simulink model "OIRT"  (Simulink 8.5)
settings: Solver=ode3  SolverMode=SingleTasking  StartTime=0.0  StopTime=1.0  FixedStep=2e-5  RelTol=1e-4  AbsTol=1e-6
undefined symbols (not defined in the file or in its folder): DAB, den, elements, num
libraries: powerlib x191, powerlib_extras x6
(part 3 of 9)

== system OIRT/Off-Line Analysis/Line 3/Fault ==
  faultA : Inport
  faultB : Inport  Port=2
  faultC : Inport  Port=3
  faultG : Inport  Port=4
  Tfault : Inport  Port=5
  &{,1..3} (4 alike) : Logic
  BreakerA : powerlib/Elements/Breaker  InitialState=0  SwitchingTimes="[ 1/60  5/60 ]"  External=on  BreakerResistance=0.01  SnubberResistance=1e6  SnubberCapacitance=inf  Measurements=None  MoreParameters=off  NoBreakLoop=off
  BreakerB : powerlib/Elements/Breaker  InitialState=0  SwitchingTimes="[ 1/60  5/60 ]"  External=on  BreakerResistance=0.01  SnubberResistance=1e6  SnubberCapacitance=inf  Measurements=None  MoreParameters=off  NoBreakLoop=off
  BreakerC : powerlib/Elements/Breaker  InitialState=0  SwitchingTimes="[ 1/60  5/60 ]"  External=on  BreakerResistance=0.01  SnubberResistance=1e6  SnubberCapacitance=inf  Measurements=None  MoreParameters=off  NoBreakLoop=off
  BreakerN : powerlib/Elements/Breaker  InitialState=0  SwitchingTimes="[ 1/60  5/60 ]"  External=on  BreakerResistance=0.01  SnubberResistance=1e6  SnubberCapacitance=inf  Measurements=None  MoreParameters=off  NoBreakLoop=off
  Ground : powerlib/Elements/Ground  LConnTagsString=a
  RA : powerlib/Elements/Series RLC Branch  LConnTagsString=__new0  RConnTagsString=__new0  BranchType=R  Resistance=10000  Inductance=1e-3  SetiL0=off  InitialCurrent=0  Capacitance=1e-6  Setx0=off  InitialVoltage=0  Measurements=None
  RB : powerlib/Elements/Series RLC Branch  LConnTagsString=__new0  RConnTagsString=__new0  BranchType=R  Resistance=10000  Inductance=1e-3  SetiL0=off  InitialCurrent=0  Capacitance=1e-6  Setx0=off  InitialVoltage=0  Measurements=None
  RC : powerlib/Elements/Series RLC Branch  LConnTagsString=__new0  RConnTagsString=__new0  BranchType=R  Resistance=10000  Inductance=1e-3  SetiL0=off  InitialCurrent=0  Capacitance=1e-6  Setx0=off  InitialVoltage=0  Measurements=None
  RN : powerlib/Elements/Series RLC Branch  LConnTagsString=__new0  RConnTagsString=__new0  BranchType=R  Resistance=10000  Inductance=1e-3  SetiL0=off  InitialCurrent=0  Capacitance=1e-6  Setx0=off  InitialVoltage=0  Measurements=None
  RfA : powerlib/Elements/Series RLC Branch  LConnTagsString=__new0  RConnTagsString=__new0  BranchType=R  Resistance=faultR  Inductance=1e-3  SetiL0=off  InitialCurrent=0  Capacitance=1e-6  Setx0=off  InitialVoltage=0  Measurements=None
  RfB : powerlib/Elements/Series RLC Branch  LConnTagsString=__new0  RConnTagsString=__new0  BranchType=R  Resistance=faultR  Inductance=1e-3  SetiL0=off  InitialCurrent=0  Capacitance=1e-6  Setx0=off  InitialVoltage=0  Measurements=None
  RfC : powerlib/Elements/Series RLC Branch  LConnTagsString=__new0  RConnTagsString=__new0  BranchType=R  Resistance=faultR  Inductance=1e-3  SetiL0=off  InitialCurrent=0  Capacitance=1e-6  Setx0=off  InitialVoltage=0  Measurements=None
  A : PMIOPort  Tag=PMCPort  Port=1  Side=Left
  B : PMIOPort  Tag=PMCPort  Port=2  Side=Left
  C : PMIOPort  Tag=PMCPort  Port=3  Side=Left
  wires:
  &2/1 -> BreakerC/1
  &1/1 -> BreakerB/1
  &/1 -> BreakerA/1
  &3/1 -> BreakerN/1
  Tfault/1 -> &/2, &1/2, &2/2, &3/2
  faultG/1 -> &3/1
  faultC/1 -> &2/1
  faultB/1 -> &1/1
  faultA/1 -> &/1
  connections:
  RN/RConn1 -- Ground/LConn1 -- BreakerN/RConn1
  RfC/RConn1 -- RfA/RConn1 -- RfB/RConn1 -- RN/LConn1 -- BreakerN/LConn1
  BreakerA/RConn1 -- RfA/LConn1 -- RA/RConn1
  BreakerB/RConn1 -- RfB/LConn1 -- RB/RConn1
  RfC/LConn1 -- RC/RConn1 -- BreakerC/RConn1
  BreakerC/LConn1 -- C/RConn1 -- RC/LConn1
  RA/LConn1 -- BreakerA/LConn1 -- A/RConn1
  BreakerB/LConn1 -- RB/LConn1 -- B/RConn1

== system OIRT/Off-Line Analysis/Line 3/Fault Selector ==
  "  " : Constant  Value=faultType
  "  +" : Logic  Operator=OR  Inputs=7
  " +" : Logic  Operator=OR  Inputs=5
  + : Logic  Operator=OR  Inputs=5
  "+ " : Logic  Operator=OR  Inputs=6
  A-B-C : Fcn  Expr=(u(1)==8)
  A-B-C-G : Fcn  Expr=(u(1)==9)
  A-G : Fcn  Expr=(u(1)==1)
  B-C : Fcn  Expr=(u(1)==4)
  B-C-G : Fcn  Expr=(u(1)==5)
  B-G : Fcn  Expr=(u(1)==2)
  C-A : Fcn  Expr=(u(1)==6)
  C-A-G : Fcn  Expr=(u(1)==7)
  C-G : Fcn  Expr=(u(1)==3)
  faultA : Outport  InitialOutput=0
  faultB : Outport  Port=2  InitialOutput=0
  faultC : Outport  Port=3  InitialOutput=0
  faultG : Outport  Port=4  InitialOutput=0
  wires:
  A-B-C/1 -> +/4, "  +"/6, " +"/4
  A-B-C-G/1 -> +/5, "+ "/6, "  +"/7, " +"/5
  C-A-G/1 -> +/3, "+ "/5, "  +"/5
  C-G/1 -> "+ "/3, "  +"/1
  B-C-G/1 -> " +"/3, "+ "/4, "  +"/3
  B-C/1 -> " +"/2, "  +"/2
  B-G/1 -> "+ "/2, " +"/1
  C-A/1 -> +/2, "  +"/4
  A-G/1 -> +/1, "+ "/1
  "+ "/1 -> faultG/1
  "  +"/1 -> faultC/1
  " +"/1 -> faultB/1
  +/1 -> faultA/1
  "  "/1 -> B-C-G/1, A-B-C-G/1, A-B-C/1, C-A-G/1, C-A/1, B-C/1, B-G/1, A-G/1, C-G/1

== system OIRT/On-Line Analysis/Line 1/Fault ==
  faultA : Inport
  faultB : Inport  Port=2
  faultC : Inport  Port=3
  faultG : Inport  Port=4
  Tfault : Inport  Port=5
  &{,1..3} (4 alike) : Logic
  BreakerA : powerlib/Elements/Breaker  InitialState=0  SwitchingTimes="[ 1/60  5/60 ]"  External=on  BreakerResistance=0.01  SnubberResistance=1e6  SnubberCapacitance=inf  Measurements=None  MoreParameters=off  NoBreakLoop=off
  BreakerB : powerlib/Elements/Breaker  InitialState=0  SwitchingTimes="[ 1/60  5/60 ]"  External=on  BreakerResistance=0.01  SnubberResistance=1e6  SnubberCapacitance=inf  Measurements=None  MoreParameters=off  NoBreakLoop=off
  BreakerC : powerlib/Elements/Breaker  InitialState=0  SwitchingTimes="[ 1/60  5/60 ]"  External=on  BreakerResistance=0.01  SnubberResistance=1e6  SnubberCapacitance=inf  Measurements=None  MoreParameters=off  NoBreakLoop=off
  BreakerN : powerlib/Elements/Breaker  InitialState=0  SwitchingTimes="[ 1/60  5/60 ]"  External=on  BreakerResistance=0.01  SnubberResistance=1e6  SnubberCapacitance=inf  Measurements=None  MoreParameters=off  NoBreakLoop=off
  Ground : powerlib/Elements/Ground  LConnTagsString=a
  RA : powerlib/Elements/Series RLC Branch  LConnTagsString=__new0  RConnTagsString=__new0  BranchType=R  Resistance=10000  Inductance=1e-3  SetiL0=off  InitialCurrent=0  Capacitance=1e-6  Setx0=off  InitialVoltage=0  Measurements=None
  RB : powerlib/Elements/Series RLC Branch  LConnTagsString=__new0  RConnTagsString=__new0  BranchType=R  Resistance=10000  Inductance=1e-3  SetiL0=off  InitialCurrent=0  Capacitance=1e-6  Setx0=off  InitialVoltage=0  Measurements=None
  RC : powerlib/Elements/Series RLC Branch  LConnTagsString=__new0  RConnTagsString=__new0  BranchType=R  Resistance=10000  Inductance=1e-3  SetiL0=off  InitialCurrent=0  Capacitance=1e-6  Setx0=off  InitialVoltage=0  Measurements=None
  RN : powerlib/Elements/Series RLC Branch  LConnTagsString=__new0  RConnTagsString=__new0  BranchType=R  Resistance=10000  Inductance=1e-3  SetiL0=off  InitialCurrent=0  Capacitance=1e-6  Setx0=off  InitialVoltage=0  Measurements=None
  RfA : powerlib/Elements/Series RLC Branch  LConnTagsString=__new0  RConnTagsString=__new0  BranchType=R  Resistance=faultR  Inductance=1e-3  SetiL0=off  InitialCurrent=0  Capacitance=1e-6  Setx0=off  InitialVoltage=0  Measurements=None
  RfB : powerlib/Elements/Series RLC Branch  LConnTagsString=__new0  RConnTagsString=__new0  BranchType=R  Resistance=faultR  Inductance=1e-3  SetiL0=off  InitialCurrent=0  Capacitance=1e-6  Setx0=off  InitialVoltage=0  Measurements=None
  RfC : powerlib/Elements/Series RLC Branch  LConnTagsString=__new0  RConnTagsString=__new0  BranchType=R  Resistance=faultR  Inductance=1e-3  SetiL0=off  InitialCurrent=0  Capacitance=1e-6  Setx0=off  InitialVoltage=0  Measurements=None
  A : PMIOPort  Tag=PMCPort  Port=1  Side=Left
  B : PMIOPort  Tag=PMCPort  Port=2  Side=Left
  C : PMIOPort  Tag=PMCPort  Port=3  Side=Left
  wires:
  faultA/1 -> &/1
  faultB/1 -> &1/1
  faultC/1 -> &2/1
  faultG/1 -> &3/1
  Tfault/1 -> &3/2, &2/2, &1/2, &/2
  &3/1 -> BreakerN/1
  &/1 -> BreakerA/1
  &1/1 -> BreakerB/1
  &2/1 -> BreakerC/1
  connections:
  B/RConn1 -- RB/LConn1 -- BreakerB/LConn1
  A/RConn1 -- BreakerA/LConn1 -- RA/LConn1
  RC/LConn1 -- C/RConn1 -- BreakerC/LConn1
  BreakerC/RConn1 -- RC/RConn1 -- RfC/LConn1
  RB/RConn1 -- RfB/LConn1 -- BreakerB/RConn1
  RA/RConn1 -- RfA/LConn1 -- BreakerA/RConn1
  BreakerN/LConn1 -- RN/LConn1 -- RfB/RConn1 -- RfA/RConn1 -- RfC/RConn1
  BreakerN/RConn1 -- Ground/LConn1 -- RN/RConn1

== system OIRT/On-Line Analysis/Line 1/Fault Selector ==
  "  " : Constant  Value=faultType
  "  +" : Logic  Operator=OR  Inputs=7
  " +" : Logic  Operator=OR  Inputs=5
  + : Logic  Operator=OR  Inputs=5
  "+ " : Logic  Operator=OR  Inputs=6
  A-B-C : Fcn  Expr=(u(1)==8)
  A-B-C-G : Fcn  Expr=(u(1)==9)
  A-G : Fcn  Expr=(u(1)==1)
  B-C : Fcn  Expr=(u(1)==4)
  B-C-G : Fcn  Expr=(u(1)==5)
  B-G : Fcn  Expr=(u(1)==2)
  C-A : Fcn  Expr=(u(1)==6)
  C-A-G : Fcn  Expr=(u(1)==7)
  C-G : Fcn  Expr=(u(1)==3)
  faultA : Outport  InitialOutput=0
  faultB : Outport  Port=2  InitialOutput=0
  faultC : Outport  Port=3  InitialOutput=0
  faultG : Outport  Port=4  InitialOutput=0
  wires:
  "  "/1 -> C-G/1, A-G/1, B-G/1, B-C/1, C-A/1, C-A-G/1, A-B-C/1, A-B-C-G/1, B-C-G/1
  +/1 -> faultA/1
  " +"/1 -> faultB/1
  "  +"/1 -> faultC/1
  "+ "/1 -> faultG/1
  A-G/1 -> "+ "/1, +/1
  C-A/1 -> "  +"/4, +/2
  B-G/1 -> " +"/1, "+ "/2
  B-C/1 -> "  +"/2, " +"/2
  B-C-G/1 -> "  +"/3, "+ "/4, " +"/3
  C-G/1 -> "  +"/1, "+ "/3
  C-A-G/1 -> "  +"/5, "+ "/5, +/3
  A-B-C-G/1 -> " +"/5, "  +"/7, "+ "/6, +/5
  A-B-C/1 -> " +"/4, "  +"/6, +/4

== system OIRT/On-Line Analysis/Line 2/Fault ==
  faultA : Inport
  faultB : Inport  Port=2
  faultC : Inport  Port=3
  faultG : Inport  Port=4
  Tfault : Inport  Port=5
  &{,1..3} (4 alike) : Logic
  BreakerA : powerlib/Elements/Breaker  InitialState=0  SwitchingTimes="[ 1/60  5/60 ]"  External=on  BreakerResistance=0.01  SnubberResistance=1e6  SnubberCapacitance=inf  Measurements=None  MoreParameters=off  NoBreakLoop=off
  BreakerB : powerlib/Elements/Breaker  InitialState=0  SwitchingTimes="[ 1/60  5/60 ]"  External=on  BreakerResistance=0.01  SnubberResistance=1e6  SnubberCapacitance=inf  Measurements=None  MoreParameters=off  NoBreakLoop=off
  BreakerC : powerlib/Elements/Breaker  InitialState=0  SwitchingTimes="[ 1/60  5/60 ]"  External=on  BreakerResistance=0.01  SnubberResistance=1e6  SnubberCapacitance=inf  Measurements=None  MoreParameters=off  NoBreakLoop=off
  BreakerN : powerlib/Elements/Breaker  InitialState=0  SwitchingTimes="[ 1/60  5/60 ]"  External=on  BreakerResistance=0.01  SnubberResistance=1e6  SnubberCapacitance=inf  Measurements=None  MoreParameters=off  NoBreakLoop=off
  Ground : powerlib/Elements/Ground  LConnTagsString=a
  RA : powerlib/Elements/Series RLC Branch  LConnTagsString=__new0  RConnTagsString=__new0  BranchType=R  Resistance=10000  Inductance=1e-3  SetiL0=off  InitialCurrent=0  Capacitance=1e-6  Setx0=off  InitialVoltage=0  Measurements=None
  RB : powerlib/Elements/Series RLC Branch  LConnTagsString=__new0  RConnTagsString=__new0  BranchType=R  Resistance=10000  Inductance=1e-3  SetiL0=off  InitialCurrent=0  Capacitance=1e-6  Setx0=off  InitialVoltage=0  Measurements=None
  RC : powerlib/Elements/Series RLC Branch  LConnTagsString=__new0  RConnTagsString=__new0  BranchType=R  Resistance=10000  Inductance=1e-3  SetiL0=off  InitialCurrent=0  Capacitance=1e-6  Setx0=off  InitialVoltage=0  Measurements=None
  RN : powerlib/Elements/Series RLC Branch  LConnTagsString=__new0  RConnTagsString=__new0  BranchType=R  Resistance=10000  Inductance=1e-3  SetiL0=off  InitialCurrent=0  Capacitance=1e-6  Setx0=off  InitialVoltage=0  Measurements=None
  RfA : powerlib/Elements/Series RLC Branch  LConnTagsString=__new0  RConnTagsString=__new0  BranchType=R  Resistance=faultR  Inductance=1e-3  SetiL0=off  InitialCurrent=0  Capacitance=1e-6  Setx0=off  InitialVoltage=0  Measurements=None
  RfB : powerlib/Elements/Series RLC Branch  LConnTagsString=__new0  RConnTagsString=__new0  BranchType=R  Resistance=faultR  Inductance=1e-3  SetiL0=off  InitialCurrent=0  Capacitance=1e-6  Setx0=off  InitialVoltage=0  Measurements=None
  RfC : powerlib/Elements/Series RLC Branch  LConnTagsString=__new0  RConnTagsString=__new0  BranchType=R  Resistance=faultR  Inductance=1e-3  SetiL0=off  InitialCurrent=0  Capacitance=1e-6  Setx0=off  InitialVoltage=0  Measurements=None
  A : PMIOPort  Tag=PMCPort  Port=1  Side=Left
  B : PMIOPort  Tag=PMCPort  Port=2  Side=Left
  C : PMIOPort  Tag=PMCPort  Port=3  Side=Left
  wires:
  faultA/1 -> &/1
  faultB/1 -> &1/1
  faultC/1 -> &2/1
  faultG/1 -> &3/1
  Tfault/1 -> &3/2, &2/2, &1/2, &/2
  &3/1 -> BreakerN/1
  &/1 -> BreakerA/1
  &1/1 -> BreakerB/1
  &2/1 -> BreakerC/1
  connections:
  B/RConn1 -- RB/LConn1 -- BreakerB/LConn1
  A/RConn1 -- BreakerA/LConn1 -- RA/LConn1
  RC/LConn1 -- C/RConn1 -- BreakerC/LConn1
  BreakerC/RConn1 -- RC/RConn1 -- RfC/LConn1
  RB/RConn1 -- RfB/LConn1 -- BreakerB/RConn1
  RA/RConn1 -- RfA/LConn1 -- BreakerA/RConn1
  BreakerN/LConn1 -- RN/LConn1 -- RfB/RConn1 -- RfA/RConn1 -- RfC/RConn1
  BreakerN/RConn1 -- Ground/LConn1 -- RN/RConn1

== system OIRT/On-Line Analysis/Line 2/Fault Selector ==
  "  " : Constant  Value=faultType
  "  +" : Logic  Operator=OR  Inputs=7
  " +" : Logic  Operator=OR  Inputs=5
  + : Logic  Operator=OR  Inputs=5
  "+ " : Logic  Operator=OR  Inputs=6
  A-B-C : Fcn  Expr=(u(1)==8)
  A-B-C-G : Fcn  Expr=(u(1)==9)
  A-G : Fcn  Expr=(u(1)==1)
  B-C : Fcn  Expr=(u(1)==4)
  B-C-G : Fcn  Expr=(u(1)==5)
  B-G : Fcn  Expr=(u(1)==2)
  C-A : Fcn  Expr=(u(1)==6)
  C-A-G : Fcn  Expr=(u(1)==7)
  C-G : Fcn  Expr=(u(1)==3)
  faultA : Outport  InitialOutput=0
  faultB : Outport  Port=2  InitialOutput=0
  faultC : Outport  Port=3  InitialOutput=0
  faultG : Outport  Port=4  InitialOutput=0
  wires:
  "  "/1 -> C-G/1, A-G/1, B-G/1, B-C/1, C-A/1, C-A-G/1, A-B-C/1, A-B-C-G/1, B-C-G/1
  +/1 -> faultA/1
  " +"/1 -> faultB/1
  "  +"/1 -> faultC/1
  "+ "/1 -> faultG/1
  A-G/1 -> "+ "/1, +/1
  C-A/1 -> "  +"/4, +/2
  B-G/1 -> " +"/1, "+ "/2
  B-C/1 -> "  +"/2, " +"/2
  B-C-G/1 -> "  +"/3, "+ "/4, " +"/3
  C-G/1 -> "  +"/1, "+ "/3
  C-A-G/1 -> "  +"/5, "+ "/5, +/3
  A-B-C-G/1 -> " +"/5, "  +"/7, "+ "/6, +/5
  A-B-C/1 -> " +"/4, "  +"/6, +/4

== system OIRT/On-Line Analysis/Line 3/Fault ==
  faultA : Inport
  faultB : Inport  Port=2
  faultC : Inport  Port=3
  faultG : Inport  Port=4
  Tfault : Inport  Port=5
  &{,1..3} (4 alike) : Logic
  BreakerA : powerlib/Elements/Breaker  InitialState=0  SwitchingTimes="[ 1/60  5/60 ]"  External=on  BreakerResistance=0.01  SnubberResistance=1e6  SnubberCapacitance=inf  Measurements=None  MoreParameters=off  NoBreakLoop=off
  BreakerB : powerlib/Elements/Breaker  InitialState=0  SwitchingTimes="[ 1/60  5/60 ]"  External=on  BreakerResistance=0.01  SnubberResistance=1e6  SnubberCapacitance=inf  Measurements=None  MoreParameters=off  NoBreakLoop=off
  BreakerC : powerlib/Elements/Breaker  InitialState=0  SwitchingTimes="[ 1/60  5/60 ]"  External=on  BreakerResistance=0.01  SnubberResistance=1e6  SnubberCapacitance=inf  Measurements=None  MoreParameters=off  NoBreakLoop=off
  BreakerN : powerlib/Elements/Breaker  InitialState=0  SwitchingTimes="[ 1/60  5/60 ]"  External=on  BreakerResistance=0.01  SnubberResistance=1e6  SnubberCapacitance=inf  Measurements=None  MoreParameters=off  NoBreakLoop=off
  Ground : powerlib/Elements/Ground  LConnTagsString=a
  RA : powerlib/Elements/Series RLC Branch  LConnTagsString=__new0  RConnTagsString=__new0  BranchType=R  Resistance=10000  Inductance=1e-3  SetiL0=off  InitialCurrent=0  Capacitance=1e-6  Setx0=off  InitialVoltage=0  Measurements=None
  RB : powerlib/Elements/Series RLC Branch  LConnTagsString=__new0  RConnTagsString=__new0  BranchType=R  Resistance=10000  Inductance=1e-3  SetiL0=off  InitialCurrent=0  Capacitance=1e-6  Setx0=off  InitialVoltage=0  Measurements=None
  RC : powerlib/Elements/Series RLC Branch  LConnTagsString=__new0  RConnTagsString=__new0  BranchType=R  Resistance=10000  Inductance=1e-3  SetiL0=off  InitialCurrent=0  Capacitance=1e-6  Setx0=off  InitialVoltage=0  Measurements=None
  RN : powerlib/Elements/Series RLC Branch  LConnTagsString=__new0  RConnTagsString=__new0  BranchType=R  Resistance=10000  Inductance=1e-3  SetiL0=off  InitialCurrent=0  Capacitance=1e-6  Setx0=off  InitialVoltage=0  Measurements=None
  RfA : powerlib/Elements/Series RLC Branch  LConnTagsString=__new0  RConnTagsString=__new0  BranchType=R  Resistance=faultR  Inductance=1e-3  SetiL0=off  InitialCurrent=0  Capacitance=1e-6  Setx0=off  InitialVoltage=0  Measurements=None
  RfB : powerlib/Elements/Series RLC Branch  LConnTagsString=__new0  RConnTagsString=__new0  BranchType=R  Resistance=faultR  Inductance=1e-3  SetiL0=off  InitialCurrent=0  Capacitance=1e-6  Setx0=off  InitialVoltage=0  Measurements=None
  RfC : powerlib/Elements/Series RLC Branch  LConnTagsString=__new0  RConnTagsString=__new0  BranchType=R  Resistance=faultR  Inductance=1e-3  SetiL0=off  InitialCurrent=0  Capacitance=1e-6  Setx0=off  InitialVoltage=0  Measurements=None
  A : PMIOPort  Tag=PMCPort  Port=1  Side=Left
  B : PMIOPort  Tag=PMCPort  Port=2  Side=Left
  C : PMIOPort  Tag=PMCPort  Port=3  Side=Left
  wires:
  &2/1 -> BreakerC/1
  &1/1 -> BreakerB/1
  &/1 -> BreakerA/1
  &3/1 -> BreakerN/1
  Tfault/1 -> &/2, &1/2, &2/2, &3/2
  faultG/1 -> &3/1
  faultC/1 -> &2/1
  faultB/1 -> &1/1
  faultA/1 -> &/1
  connections:
  RN/RConn1 -- Ground/LConn1 -- BreakerN/RConn1
  RfC/RConn1 -- RfA/RConn1 -- RfB/RConn1 -- RN/LConn1 -- BreakerN/LConn1
  BreakerA/RConn1 -- RfA/LConn1 -- RA/RConn1
  BreakerB/RConn1 -- RfB/LConn1 -- RB/RConn1
  RfC/LConn1 -- RC/RConn1 -- BreakerC/RConn1
  BreakerC/LConn1 -- C/RConn1 -- RC/LConn1
  RA/LConn1 -- BreakerA/LConn1 -- A/RConn1
  BreakerB/LConn1 -- RB/LConn1 -- B/RConn1

== system OIRT/On-Line Analysis/Line 3/Fault Selector ==
  "  " : Constant  Value=faultType
  "  +" : Logic  Operator=OR  Inputs=7
  " +" : Logic  Operator=OR  Inputs=5
  + : Logic  Operator=OR  Inputs=5
  "+ " : Logic  Operator=OR  Inputs=6
  A-B-C : Fcn  Expr=(u(1)==8)
  A-B-C-G : Fcn  Expr=(u(1)==9)
  A-G : Fcn  Expr=(u(1)==1)
  B-C : Fcn  Expr=(u(1)==4)
  B-C-G : Fcn  Expr=(u(1)==5)
  B-G : Fcn  Expr=(u(1)==2)
  C-A : Fcn  Expr=(u(1)==6)
  C-A-G : Fcn  Expr=(u(1)==7)
  C-G : Fcn  Expr=(u(1)==3)
  faultA : Outport  InitialOutput=0
  faultB : Outport  Port=2  InitialOutput=0
  faultC : Outport  Port=3  InitialOutput=0
  faultG : Outport  Port=4  InitialOutput=0
  wires:
  A-B-C/1 -> +/4, "  +"/6, " +"/4
  A-B-C-G/1 -> +/5, "+ "/6, "  +"/7, " +"/5
  C-A-G/1 -> +/3, "+ "/5, "  +"/5
  C-G/1 -> "+ "/3, "  +"/1
  B-C-G/1 -> " +"/3, "+ "/4, "  +"/3
  B-C/1 -> " +"/2, "  +"/2
  B-G/1 -> "+ "/2, " +"/1
  C-A/1 -> +/2, "  +"/4
  A-G/1 -> +/1, "+ "/1
  "+ "/1 -> faultG/1
  "  +"/1 -> faultC/1
  " +"/1 -> faultB/1
  +/1 -> faultA/1
  "  "/1 -> B-C-G/1, A-B-C-G/1, A-B-C/1, C-A-G/1, C-A/1, B-C/1, B-G/1, A-G/1, C-G/1

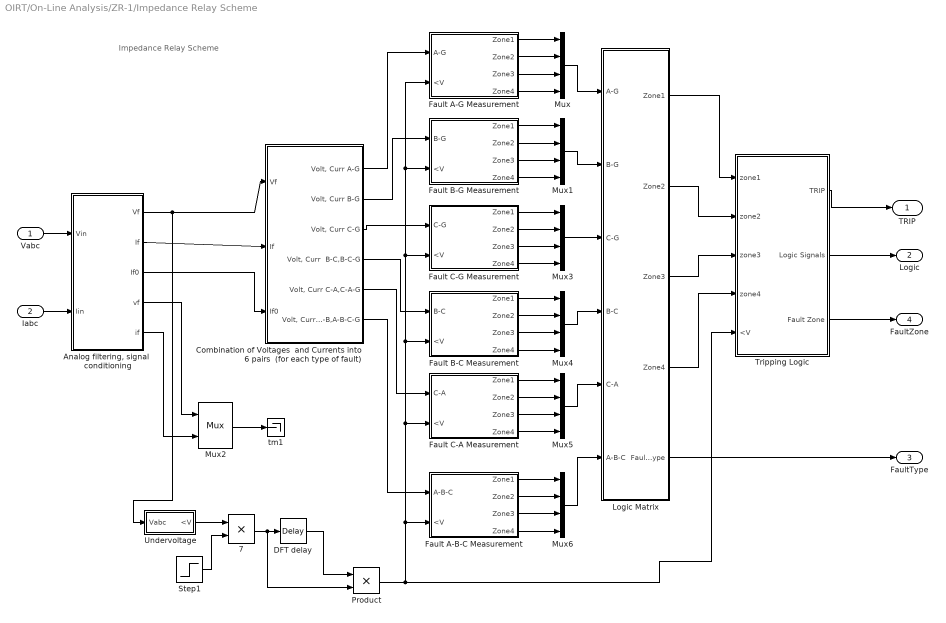
== system OIRT/On-Line Analysis/ZR-1/Impedance Relay Scheme ==
  note: Impedance Relay Scheme
  Vabc : Inport
  Iabc : Inport  Port=2
  " 7" : Product  RndMeth=Zero
  "Analog filtering, signal  conditioning" : Subsystem
  Combination of Voltages  and Currents into 6 pairs  (for each type of fault) : Subsystem
  DFT delay : TransportDelay  DelayTime=0.017  BufferSize=30720
  Fault A-B-C Measurement : Subsystem
  Fault A-G Measurement : Subsystem
  Fault B-C Measurement : Subsystem
  Fault B-G Measurement : Subsystem
  Fault C-A Measurement : Subsystem
  Fault C-G Measurement : Subsystem
  Logic Matrix : Subsystem
  Mux{,1,3..6} (6 alike) : Mux
  Mux2 : Mux  Inputs=2
  Product : Product  RndMeth=Zero
  Step1 : Step  Time=0.017  SampleTime=0
  Tripping Logic : Subsystem
  Undervoltage : Subsystem
  tm1 : Terminator
  "TRIP " : Outport  InitialOutput=0
  Logic : Outport  Port=2  InitialOutput=0
  FaultType : Outport  Port=3  InitialOutput=0
  FaultZone : Outport  Port=4  InitialOutput=0
  wires:
  Mux2/1 -> tm1/1
  Tripping Logic/3(Fault Zone) -> FaultZone/1
  Product/1 -> Tripping Logic/5(<V), Fault A-B-C Measurement/2(<V), Fault C-A Measurement/2(<V), Fault B-C Measurement/2(<V), Fault C-G Measurement/2(<V), Fault B-G Measurement/2(<V), Fault A-G Measurement/2(<V)
  Logic Matrix/5(Fault Type) -> FaultType/1
  Tripping Logic/2(Logic Signals) -> Logic/1
  Tripping Logic/1(TRIP) -> "TRIP "/1
  Logic Matrix/4(" Zone4") -> Tripping Logic/4(zone4)
  Logic Matrix/3(" Zone3") -> Tripping Logic/3(zone3)
  Logic Matrix/2(" Zone2") -> Tripping Logic/2(zone2)
  Logic Matrix/1(" Zone1") -> Tripping Logic/1(zone1)
  Mux6/1 -> Logic Matrix/6(A-B-C)
  Mux5/1 -> Logic Matrix/5(C-A)
  Mux4/1 -> Logic Matrix/4(B-C)
  Mux3/1 -> Logic Matrix/3(C-G)
  Mux1/1 -> Logic Matrix/2(B-G)
  Mux/1 -> Logic Matrix/1(A-G)
  Fault A-B-C Measurement/4(Zone4) -> Mux6/4
  Fault A-B-C Measurement/3(Zone3) -> Mux6/3
  Fault A-B-C Measurement/2(Zone2) -> Mux6/2
  Fault A-B-C Measurement/1(Zone1) -> Mux6/1
  Fault C-A Measurement/4(Zone4) -> Mux5/4
  Fault C-A Measurement/3(Zone3) -> Mux5/3
  Fault C-A Measurement/2(Zone2) -> Mux5/2
  Fault C-A Measurement/1(Zone1) -> Mux5/1
  Fault B-C Measurement/4(Zone4) -> Mux4/4
  Fault B-C Measurement/3(Zone3) -> Mux4/3
  Fault B-C Measurement/2(Zone2) -> Mux4/2
  Fault B-C Measurement/1(Zone1) -> Mux4/1
  Fault C-G Measurement/4(Zone4) -> Mux3/4
  Fault C-G Measurement/3(Zone3) -> Mux3/3
  Fault C-G Measurement/2(Zone2) -> Mux3/2
  Fault C-G Measurement/1(Zone1) -> Mux3/1
  Fault B-G Measurement/4(Zone4) -> Mux1/4
  Fault B-G Measurement/3(Zone3) -> Mux1/3
  Fault B-G Measurement/2(Zone2) -> Mux1/2
  Fault B-G Measurement/1(Zone1) -> Mux1/1
  Fault A-G Measurement/4(Zone4) -> Mux/4
  Fault A-G Measurement/3(Zone3) -> Mux/3
  Fault A-G Measurement/2(Zone2) -> Mux/2
  Fault A-G Measurement/1(Zone1) -> Mux/1
  DFT delay/1 -> Product/1
  Combination of Voltages  and Currents into 6 pairs  (for each type of fault)/6("Volt, Curr A-B,A-B-C-G") -> Fault A-B-C Measurement/1(A-B-C)
  Combination of Voltages  and Currents into 6 pairs  (for each type of fault)/5("Volt, Curr C-A,C-A-G") -> Fault C-A Measurement/1(C-A)
  Combination of Voltages  and Currents into 6 pairs  (for each type of fault)/4("Volt, Curr  B-C,B-C-G") -> Fault B-C Measurement/1(B-C)
  Combination of Voltages  and Currents into 6 pairs  (for each type of fault)/3("Volt, Curr C-G") -> Fault C-G Measurement/1(C-G)
  Combination of Voltages  and Currents into 6 pairs  (for each type of fault)/2("Volt, Curr B-G") -> Fault B-G Measurement/1(B-G)
  "Analog filtering, signal  conditioning"/3(If0) -> Combination of Voltages  and Currents into 6 pairs  (for each type of fault)/3(If0)
  "Analog filtering, signal  conditioning"/2(If) -> Combination of Voltages  and Currents into 6 pairs  (for each type of fault)/2(If)
  "Analog filtering, signal  conditioning"/5(if) -> Mux2/2
  "Analog filtering, signal  conditioning"/4(vf) -> Mux2/1
  "Analog filtering, signal  conditioning"/1(Vf) -> Undervoltage/1("Vabc  "), Combination of Voltages  and Currents into 6 pairs  (for each type of fault)/1(Vf)
  " 7"/1 -> Product/2, DFT delay/1
  Step1/1 -> " 7"/2
  Undervoltage/1(<V) -> " 7"/1
  Combination of Voltages  and Currents into 6 pairs  (for each type of fault)/1("Volt, Curr A-G") -> Fault A-G Measurement/1(A-G)
  Iabc/1 -> "Analog filtering, signal  conditioning"/2(Iin)
  Vabc/1 -> "Analog filtering, signal  conditioning"/1(Vin)

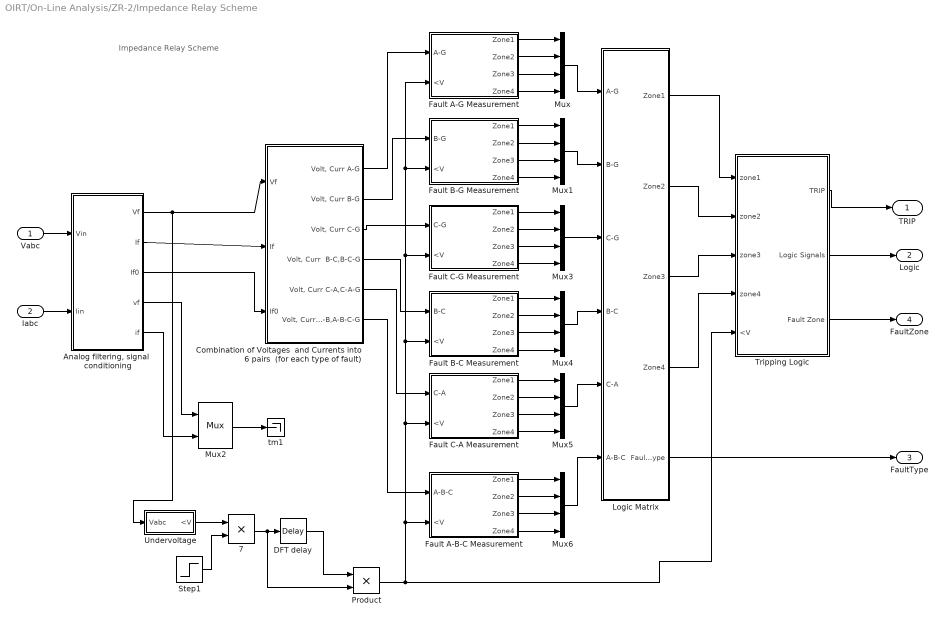
== system OIRT/On-Line Analysis/ZR-2/Impedance Relay Scheme ==
  note: Impedance Relay Scheme
  Vabc : Inport
  Iabc : Inport  Port=2
  " 7" : Product  RndMeth=Zero
  "Analog filtering, signal  conditioning" : Subsystem
  Combination of Voltages  and Currents into 6 pairs  (for each type of fault) : Subsystem
  DFT delay : TransportDelay  DelayTime=0.017  BufferSize=30720
  Fault A-B-C Measurement : Subsystem
  Fault A-G Measurement : Subsystem
  Fault B-C Measurement : Subsystem
  Fault B-G Measurement : Subsystem
  Fault C-A Measurement : Subsystem
  Fault C-G Measurement : Subsystem
  Logic Matrix : Subsystem
  Mux{,1,3..6} (6 alike) : Mux
  Mux2 : Mux  Inputs=2
  Product : Product  RndMeth=Zero
  Step1 : Step  Time=0.017  SampleTime=0
  Tripping Logic : Subsystem
  Undervoltage : Subsystem
  tm1 : Terminator
  "TRIP " : Outport  InitialOutput=0
  Logic : Outport  Port=2  InitialOutput=0
  FaultType : Outport  Port=3  InitialOutput=0
  FaultZone : Outport  Port=4  InitialOutput=0
  wires:
  Mux2/1 -> tm1/1
  Tripping Logic/3(Fault Zone) -> FaultZone/1
  Product/1 -> Tripping Logic/5(<V), Fault A-B-C Measurement/2(<V), Fault C-A Measurement/2(<V), Fault B-C Measurement/2(<V), Fault C-G Measurement/2(<V), Fault B-G Measurement/2(<V), Fault A-G Measurement/2(<V)
  Logic Matrix/5(Fault Type) -> FaultType/1
  Tripping Logic/2(Logic Signals) -> Logic/1
  Tripping Logic/1(TRIP) -> "TRIP "/1
  Logic Matrix/4(" Zone4") -> Tripping Logic/4(zone4)
  Logic Matrix/3(" Zone3") -> Tripping Logic/3(zone3)
  Logic Matrix/2(" Zone2") -> Tripping Logic/2(zone2)
  Logic Matrix/1(" Zone1") -> Tripping Logic/1(zone1)
  Mux6/1 -> Logic Matrix/6(A-B-C)
  Mux5/1 -> Logic Matrix/5(C-A)
  Mux4/1 -> Logic Matrix/4(B-C)
  Mux3/1 -> Logic Matrix/3(C-G)
  Mux1/1 -> Logic Matrix/2(B-G)
  Mux/1 -> Logic Matrix/1(A-G)
  Fault A-B-C Measurement/4(Zone4) -> Mux6/4
  Fault A-B-C Measurement/3(Zone3) -> Mux6/3
  Fault A-B-C Measurement/2(Zone2) -> Mux6/2
  Fault A-B-C Measurement/1(Zone1) -> Mux6/1
  Fault C-A Measurement/4(Zone4) -> Mux5/4
  Fault C-A Measurement/3(Zone3) -> Mux5/3
  Fault C-A Measurement/2(Zone2) -> Mux5/2
  Fault C-A Measurement/1(Zone1) -> Mux5/1
  Fault B-C Measurement/4(Zone4) -> Mux4/4
  Fault B-C Measurement/3(Zone3) -> Mux4/3
  Fault B-C Measurement/2(Zone2) -> Mux4/2
  Fault B-C Measurement/1(Zone1) -> Mux4/1
  Fault C-G Measurement/4(Zone4) -> Mux3/4
  Fault C-G Measurement/3(Zone3) -> Mux3/3
  Fault C-G Measurement/2(Zone2) -> Mux3/2
  Fault C-G Measurement/1(Zone1) -> Mux3/1
  Fault B-G Measurement/4(Zone4) -> Mux1/4
  Fault B-G Measurement/3(Zone3) -> Mux1/3
  Fault B-G Measurement/2(Zone2) -> Mux1/2
  Fault B-G Measurement/1(Zone1) -> Mux1/1
  Fault A-G Measurement/4(Zone4) -> Mux/4
  Fault A-G Measurement/3(Zone3) -> Mux/3
  Fault A-G Measurement/2(Zone2) -> Mux/2
  Fault A-G Measurement/1(Zone1) -> Mux/1
  DFT delay/1 -> Product/1
  Combination of Voltages  and Currents into 6 pairs  (for each type of fault)/6("Volt, Curr A-B,A-B-C-G") -> Fault A-B-C Measurement/1(A-B-C)
  Combination of Voltages  and Currents into 6 pairs  (for each type of fault)/5("Volt, Curr C-A,C-A-G") -> Fault C-A Measurement/1(C-A)
  Combination of Voltages  and Currents into 6 pairs  (for each type of fault)/4("Volt, Curr  B-C,B-C-G") -> Fault B-C Measurement/1(B-C)
  Combination of Voltages  and Currents into 6 pairs  (for each type of fault)/3("Volt, Curr C-G") -> Fault C-G Measurement/1(C-G)
  Combination of Voltages  and Currents into 6 pairs  (for each type of fault)/2("Volt, Curr B-G") -> Fault B-G Measurement/1(B-G)
  "Analog filtering, signal  conditioning"/3(If0) -> Combination of Voltages  and Currents into 6 pairs  (for each type of fault)/3(If0)
  "Analog filtering, signal  conditioning"/2(If) -> Combination of Voltages  and Currents into 6 pairs  (for each type of fault)/2(If)
  "Analog filtering, signal  conditioning"/5(if) -> Mux2/2
  "Analog filtering, signal  conditioning"/4(vf) -> Mux2/1
  "Analog filtering, signal  conditioning"/1(Vf) -> Undervoltage/1("Vabc  "), Combination of Voltages  and Currents into 6 pairs  (for each type of fault)/1(Vf)
  " 7"/1 -> Product/2, DFT delay/1
  Step1/1 -> " 7"/2
  Undervoltage/1(<V) -> " 7"/1
  Combination of Voltages  and Currents into 6 pairs  (for each type of fault)/1("Volt, Curr A-G") -> Fault A-G Measurement/1(A-G)
  Iabc/1 -> "Analog filtering, signal  conditioning"/2(Iin)
  Vabc/1 -> "Analog filtering, signal  conditioning"/1(Vin)

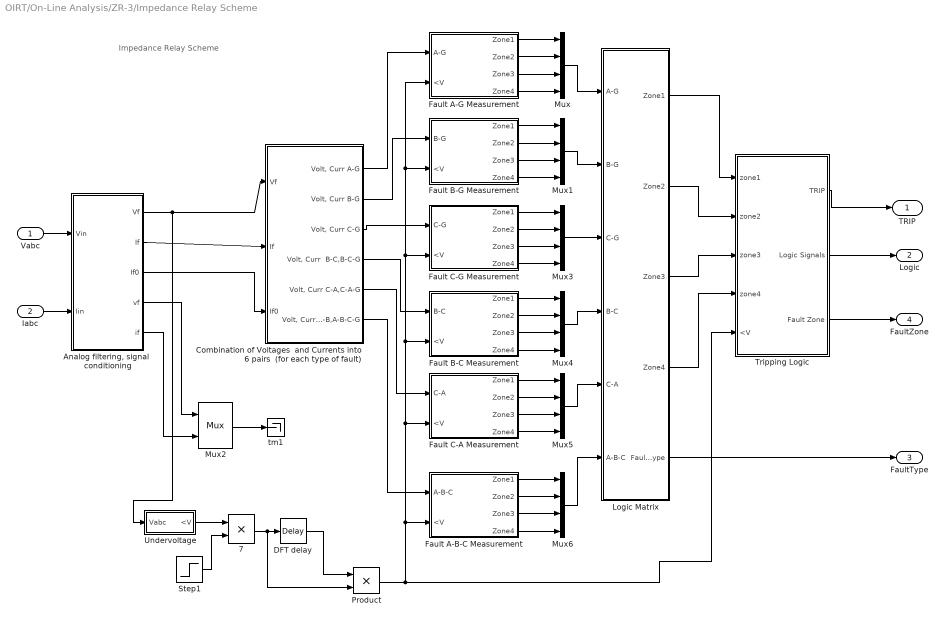
== system OIRT/On-Line Analysis/ZR-3/Impedance Relay Scheme ==
  note: Impedance Relay Scheme
  Vabc : Inport
  Iabc : Inport  Port=2
  " 7" : Product  RndMeth=Zero
  "Analog filtering, signal  conditioning" : Subsystem
  Combination of Voltages  and Currents into 6 pairs  (for each type of fault) : Subsystem
  DFT delay : TransportDelay  DelayTime=0.017  BufferSize=30720
  Fault A-B-C Measurement : Subsystem
  Fault A-G Measurement : Subsystem
  Fault B-C Measurement : Subsystem
  Fault B-G Measurement : Subsystem
  Fault C-A Measurement : Subsystem
  Fault C-G Measurement : Subsystem
  Logic Matrix : Subsystem
  Mux{,1,3..6} (6 alike) : Mux
  Mux2 : Mux  Inputs=2
  Product : Product  RndMeth=Zero
  Step1 : Step  Time=0.017  SampleTime=0
  Tripping Logic : Subsystem
  Undervoltage : Subsystem
  tm1 : Terminator
  "TRIP " : Outport  InitialOutput=0
  Logic : Outport  Port=2  InitialOutput=0
  FaultType : Outport  Port=3  InitialOutput=0
  FaultZone : Outport  Port=4  InitialOutput=0
  wires:
  Vabc/1 -> "Analog filtering, signal  conditioning"/1(Vin)
  Iabc/1 -> "Analog filtering, signal  conditioning"/2(Iin)
  Combination of Voltages  and Currents into 6 pairs  (for each type of fault)/1("Volt, Curr A-G") -> Fault A-G Measurement/1(A-G)
  Undervoltage/1(<V) -> " 7"/1
  Step1/1 -> " 7"/2
  " 7"/1 -> DFT delay/1, Product/2
  "Analog filtering, signal  conditioning"/1(Vf) -> Combination of Voltages  and Currents into 6 pairs  (for each type of fault)/1(Vf), Undervoltage/1("Vabc  ")
  "Analog filtering, signal  conditioning"/4(vf) -> Mux2/1
  "Analog filtering, signal  conditioning"/5(if) -> Mux2/2
  "Analog filtering, signal  conditioning"/2(If) -> Combination of Voltages  and Currents into 6 pairs  (for each type of fault)/2(If)
  "Analog filtering, signal  conditioning"/3(If0) -> Combination of Voltages  and Currents into 6 pairs  (for each type of fault)/3(If0)
  Combination of Voltages  and Currents into 6 pairs  (for each type of fault)/2("Volt, Curr B-G") -> Fault B-G Measurement/1(B-G)
  Combination of Voltages  and Currents into 6 pairs  (for each type of fault)/3("Volt, Curr C-G") -> Fault C-G Measurement/1(C-G)
  Combination of Voltages  and Currents into 6 pairs  (for each type of fault)/4("Volt, Curr  B-C,B-C-G") -> Fault B-C Measurement/1(B-C)
  Combination of Voltages  and Currents into 6 pairs  (for each type of fault)/5("Volt, Curr C-A,C-A-G") -> Fault C-A Measurement/1(C-A)
  Combination of Voltages  and Currents into 6 pairs  (for each type of fault)/6("Volt, Curr A-B,A-B-C-G") -> Fault A-B-C Measurement/1(A-B-C)
  DFT delay/1 -> Product/1
  Fault A-G Measurement/1(Zone1) -> Mux/1
  Fault A-G Measurement/2(Zone2) -> Mux/2
  Fault A-G Measurement/3(Zone3) -> Mux/3
  Fault A-G Measurement/4(Zone4) -> Mux/4
  Fault B-G Measurement/1(Zone1) -> Mux1/1
  Fault B-G Measurement/2(Zone2) -> Mux1/2
  Fault B-G Measurement/3(Zone3) -> Mux1/3
  Fault B-G Measurement/4(Zone4) -> Mux1/4
  Fault C-G Measurement/1(Zone1) -> Mux3/1
  Fault C-G Measurement/2(Zone2) -> Mux3/2
  Fault C-G Measurement/3(Zone3) -> Mux3/3
  Fault C-G Measurement/4(Zone4) -> Mux3/4
  Fault B-C Measurement/1(Zone1) -> Mux4/1
  Fault B-C Measurement/2(Zone2) -> Mux4/2
  Fault B-C Measurement/3(Zone3) -> Mux4/3
  Fault B-C Measurement/4(Zone4) -> Mux4/4
  Fault C-A Measurement/1(Zone1) -> Mux5/1
  Fault C-A Measurement/2(Zone2) -> Mux5/2
  Fault C-A Measurement/3(Zone3) -> Mux5/3
  Fault C-A Measurement/4(Zone4) -> Mux5/4
  Fault A-B-C Measurement/1(Zone1) -> Mux6/1
  Fault A-B-C Measurement/2(Zone2) -> Mux6/2
  Fault A-B-C Measurement/3(Zone3) -> Mux6/3
  Fault A-B-C Measurement/4(Zone4) -> Mux6/4
  Mux/1 -> Logic Matrix/1(A-G)
  Mux1/1 -> Logic Matrix/2(B-G)
  Mux3/1 -> Logic Matrix/3(C-G)
  Mux4/1 -> Logic Matrix/4(B-C)
  Mux5/1 -> Logic Matrix/5(C-A)
  Mux6/1 -> Logic Matrix/6(A-B-C)
  Logic Matrix/1(" Zone1") -> Tripping Logic/1(zone1)
  Logic Matrix/2(" Zone2") -> Tripping Logic/2(zone2)
  Logic Matrix/3(" Zone3") -> Tripping Logic/3(zone3)
  Logic Matrix/4(" Zone4") -> Tripping Logic/4(zone4)
  Tripping Logic/1(TRIP) -> "TRIP "/1
  Tripping Logic/2(Logic Signals) -> Logic/1
  Logic Matrix/5(Fault Type) -> FaultType/1
  Product/1 -> Fault A-G Measurement/2(<V), Fault B-G Measurement/2(<V), Fault C-G Measurement/2(<V), Fault B-C Measurement/2(<V), Fault C-A Measurement/2(<V), Fault A-B-C Measurement/2(<V), Tripping Logic/5(<V)
  Tripping Logic/3(Fault Zone) -> FaultZone/1
  Mux2/1 -> tm1/1

== system OIRT/On-Line Analysis/ZR-1/Impedance Relay Scheme/Analog filtering, signal  conditioning ==
  note: Acquisition Block- analog filtering,
      | signal conditioning, sampling.
  Vin : Inport
  Iin : Inport  Port=2
  CURRENTS : Subsystem
  Mux{1..4} (4 alike) : Mux  Inputs=3
  VOLTAGES : Subsystem
  Vf : Outport  InitialOutput=0
  If : Outport  Port=2  InitialOutput=0
  If0 : Outport  Port=3  InitialOutput=0
  vf : Outport  Port=4  InitialOutput=0
  if : Outport  Port=5  InitialOutput=0
  wires:
  CURRENTS/4(k0I0f) -> If0/1
  Mux4/1 -> if/1
  Mux3/1 -> If/1
  CURRENTS/7(icf) -> Mux4/3
  CURRENTS/6(ibf) -> Mux4/2
  CURRENTS/5(iaf) -> Mux4/1
  CURRENTS/3(ICf) -> Mux3/3
  CURRENTS/2(IBf) -> Mux3/2
  CURRENTS/1(IAf) -> Mux3/1
  Iin/1 -> CURRENTS/1(Iabc)
  Mux2/1 -> vf/1
  VOLTAGES/6(vcf) -> Mux2/3
  VOLTAGES/5(vbf) -> Mux2/2
  VOLTAGES/4(vaf) -> Mux2/1
  VOLTAGES/3(VCf) -> Mux1/3
  VOLTAGES/2(VBf) -> Mux1/2
  VOLTAGES/1(VAf) -> Mux1/1
  Vin/1 -> VOLTAGES/1(Vabc)
  Mux1/1 -> Vf/1

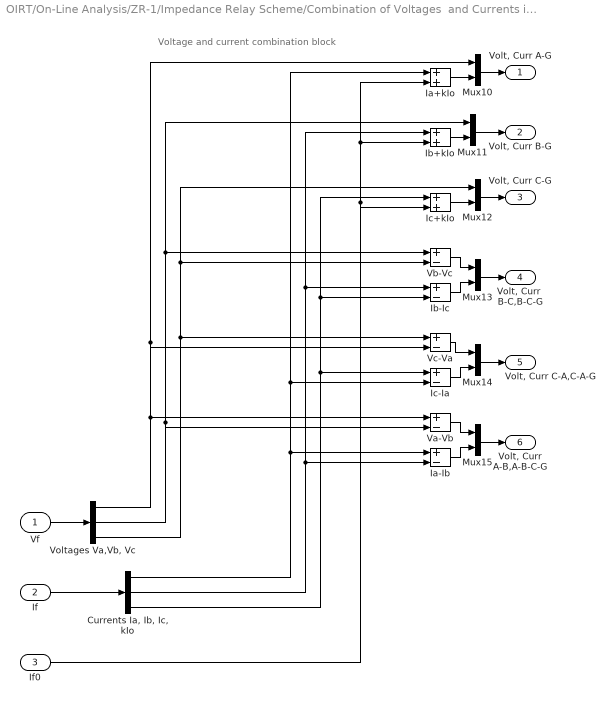
== system OIRT/On-Line Analysis/ZR-1/Impedance Relay Scheme/Combination of Voltages  and Currents into 6 pairs  (for each type of fault) ==
  note: Voltage and current combination block
  Vf : Inport
  If : Inport  Port=2
  If0 : Inport  Port=3
  "Currents Ia, Ib, Ic, kIo" : Demux  Outputs=3
  Ia+kIo : Sum  SaturateOnIntegerOverflow=on  InputSameDT=on  OutDataTypeStr=Inherit: Same as first input
  Ia-Ib : Sum  Inputs=+-  SaturateOnIntegerOverflow=on  InputSameDT=on  OutDataTypeStr=Inherit: Same as first input
  Ib+kIo : Sum  SaturateOnIntegerOverflow=on  InputSameDT=on  OutDataTypeStr=Inherit: Same as first input
  Ib-Ic : Sum  Inputs=+-  SaturateOnIntegerOverflow=on  InputSameDT=on  OutDataTypeStr=Inherit: Same as first input
  Ic+kIo : Sum  SaturateOnIntegerOverflow=on  InputSameDT=on  OutDataTypeStr=Inherit: Same as first input
  Ic-Ia : Sum  Inputs=+-  SaturateOnIntegerOverflow=on  InputSameDT=on  OutDataTypeStr=Inherit: Same as first input
  Mux{10..15} (6 alike) : Mux  Inputs=2
  Va-Vb : Sum  Inputs=+-  SaturateOnIntegerOverflow=on  InputSameDT=on  OutDataTypeStr=Inherit: Same as first input
  Vb-Vc : Sum  Inputs=+-  SaturateOnIntegerOverflow=on  InputSameDT=on  OutDataTypeStr=Inherit: Same as first input
  Vc-Va : Sum  Inputs=+-  SaturateOnIntegerOverflow=on  InputSameDT=on  OutDataTypeStr=Inherit: Same as first input
  "Voltages Va,Vb, Vc" : Demux  Outputs=3
  "Volt, Curr A-G" : Outport  InitialOutput=0
  "Volt, Curr B-G" : Outport  Port=2  InitialOutput=0
  "Volt, Curr C-G" : Outport  Port=3  InitialOutput=0
  "Volt, Curr  B-C,B-C-G" : Outport  Port=4  InitialOutput=0
  "Volt, Curr C-A,C-A-G" : Outport  Port=5  InitialOutput=0
  "Volt, Curr A-B,A-B-C-G" : Outport  Port=6  InitialOutput=0
  wires:
  If0/1 -> Ic+kIo/2, Ib+kIo/2, Ia+kIo/2
  Mux13/1 -> "Volt, Curr  B-C,B-C-G"/1
  Vb-Vc/1 -> Mux13/1
  Ib-Ic/1 -> Mux13/2
  Mux12/1 -> "Volt, Curr C-G"/1
  Ic+kIo/1 -> Mux12/2
  If/1 -> "Currents Ia, Ib, Ic, kIo"/1
  "Voltages Va,Vb, Vc"/3 -> Vc-Va/1, Vb-Vc/2, Mux12/1
  "Voltages Va,Vb, Vc"/2 -> Va-Vb/2, Vb-Vc/1, Mux11/1
  "Voltages Va,Vb, Vc"/1 -> Va-Vb/1, Vc-Va/2, Mux10/1
  Vf/1 -> "Voltages Va,Vb, Vc"/1
  Mux15/1 -> "Volt, Curr A-B,A-B-C-G"/1
  Mux14/1 -> "Volt, Curr C-A,C-A-G"/1
  Vc-Va/1 -> Mux14/1
  Mux11/1 -> "Volt, Curr B-G"/1
  Mux10/1 -> "Volt, Curr A-G"/1
  Ia+kIo/1 -> Mux10/2
  Ib+kIo/1 -> Mux11/2
  Ic-Ia/1 -> Mux14/2
  Va-Vb/1 -> Mux15/1
  Ia-Ib/1 -> Mux15/2
  "Currents Ia, Ib, Ic, kIo"/2 -> Ia-Ib/2, Ib-Ic/1, Ib+kIo/1
  "Currents Ia, Ib, Ic, kIo"/3 -> Ic-Ia/1, Ib-Ic/2, Ic+kIo/1
  "Currents Ia, Ib, Ic, kIo"/1 -> Ia-Ib/1, Ic-Ia/2, Ia+kIo/1

== system OIRT/On-Line Analysis/ZR-1/Impedance Relay Scheme/Fault A-B-C Measurement ==
  A-B-C : Inport
  <V : Inport  Port=2
  Complex to Real-Imag : ComplexToRealImag
  Impedance Module : Product  Inputs=*/  SaturateOnIntegerOverflow=on  RndMeth=Zero  InputSameDT=on  OutDataTypeStr=Inherit: Same as first input
  Mux{,1..4} (5 alike) : Mux  Inputs=2
  Voltage Current : Demux  Outputs=2
  Zone 1 : Subsystem  mask(Zone){Xr=ZoneImpedance(1)*sin(LineAngle*pi/180), Rr=ZoneImpedance(1)*cos(LineAngle*pi/180), Td=ZoneTime(1)}
      mask prompts: Xr "Reactance reach [ohm]"; Rr "Resistance reach [ohm]"; Td "Time delay [s]"
  Zone 2 : Subsystem  mask(Zone){Xr=ZoneImpedance(2)*sin(LineAngle*pi/180), Rr=ZoneImpedance(2)*cos(LineAngle*pi/180), Td=ZoneTime(2)}
      mask prompts: Xr "Reactance reach [ohm]"; Rr "Resistance reach [ohm]"; Td "Time delay [s]"
  Zone 3 : Subsystem  mask(Zone){Xr=ZoneImpedance(3)*sin(LineAngle*pi/180), Rr=ZoneImpedance(3)*cos(LineAngle*pi/180), Td=ZoneTime(3)}
      mask prompts: Xr "Reactance reach [ohm]"; Rr "Resistance reach [ohm]"; Td "Time delay [s]"
  Zone 4 : Subsystem  mask(Zone){Xr=ZoneImpedance(4)*sin(LineAngle*pi/180), Rr=ZoneImpedance(4)*cos(LineAngle*pi/180), Td=ZoneTime(4)}
      mask prompts: Xr "Reactance reach [ohm]"; Rr "Resistance reach [ohm]"; Td "Time delay [s]"
  Zone1Z : Terminator
  Zone2Z : Terminator
  Zone3Z : Terminator
  Zone4Z : Terminator
  Zone1 : Outport  InitialOutput=0
  Zone2 : Outport  Port=2  InitialOutput=0
  Zone3 : Outport  Port=3  InitialOutput=0
  Zone4 : Outport  Port=4  InitialOutput=0
  wires:
  A-B-C/1 -> Voltage Current/1
  Mux/1 -> Zone 1/1(Z), Zone 3/1(Z), Zone 4/1(Z), Zone 2/1(Z)
  Zone 1/1(TRIP) -> Zone1/1
  Zone 1/2(Zm) -> Mux1/1
  Zone 1/3(Zr) -> Mux1/2
  Zone 2/2(Zm) -> Mux2/1
  Zone 2/3(Zr) -> Mux2/2
  Zone 3/2(Zm) -> Mux3/1
  Zone 3/3(Zr) -> Mux3/2
  Zone 4/2(Zm) -> Mux4/1
  Zone 4/3(Zr) -> Mux4/2
  Zone 2/1(TRIP) -> Zone2/1
  Zone 3/1(TRIP) -> Zone3/1
  Zone 4/1(TRIP) -> Zone4/1
  Complex to Real-Imag/1 -> Mux/1
  Complex to Real-Imag/2 -> Mux/2
  <V/1 -> Zone 1/2(<V), Zone 2/2(<V), Zone 3/2(<V), Zone 4/2(<V)
  Mux1/1 -> Zone1Z/1
  Mux2/1 -> Zone2Z/1
  Mux3/1 -> Zone3Z/1
  Mux4/1 -> Zone4Z/1
  Impedance Module/1 -> Complex to Real-Imag/1
  Voltage Current/1 -> Impedance Module/1
  Voltage Current/2 -> Impedance Module/2

== system OIRT/On-Line Analysis/ZR-1/Impedance Relay Scheme/Fault A-G Measurement ==
  A-G : Inport
  <V : Inport  Port=2
  Complex to Real-Imag : ComplexToRealImag
  Impedance Module : Product  Inputs=*/  SaturateOnIntegerOverflow=on  RndMeth=Zero  InputSameDT=on  OutDataTypeStr=Inherit: Same as first input
  Mux{,1..4} (5 alike) : Mux  Inputs=2
  Voltage Current : Demux  Outputs=2
  Zone 1 : Subsystem  mask(Zone){Xr=ZoneImpedance(1)*sin(LineAngle*pi/180), Rr=ZoneImpedance(1)*cos(LineAngle*pi/180), Td=ZoneTime(1)}
      mask prompts: Xr "Reactance reach [ohm]"; Rr "Resistance reach [ohm]"; Td "Time delay [s]"
  Zone 2 : Subsystem  mask(Zone){Xr=ZoneImpedance(2)*sin(LineAngle*pi/180), Rr=ZoneImpedance(2)*cos(LineAngle*pi/180), Td=ZoneTime(2)}
      mask prompts: Xr "Reactance reach [ohm]"; Rr "Resistance reach [ohm]"; Td "Time delay [s]"
  Zone 3 : Subsystem  mask(Zone){Xr=ZoneImpedance(3)*sin(LineAngle*pi/180), Rr=ZoneImpedance(3)*cos(LineAngle*pi/180), Td=ZoneTime(3)}
      mask prompts: Xr "Reactance reach [ohm]"; Rr "Resistance reach [ohm]"; Td "Time delay [s]"
  Zone 4 : Subsystem  mask(Zone){Xr=ZoneImpedance(4)*sin(LineAngle*pi/180), Rr=ZoneImpedance(4)*cos(LineAngle*pi/180), Td=ZoneTime(4)}
      mask prompts: Xr "Reactance reach [ohm]"; Rr "Resistance reach [ohm]"; Td "Time delay [s]"
  Zone1Z : Terminator
  Zone2Z : Terminator
  Zone3Z : Terminator
  Zone4Z : Terminator
  Zone1 : Outport  InitialOutput=0
  Zone2 : Outport  Port=2  InitialOutput=0
  Zone3 : Outport  Port=3  InitialOutput=0
  Zone4 : Outport  Port=4  InitialOutput=0
  wires:
  Voltage Current/2 -> Impedance Module/2
  Voltage Current/1 -> Impedance Module/1
  Impedance Module/1 -> Complex to Real-Imag/1
  Mux4/1 -> Zone4Z/1
  Mux3/1 -> Zone3Z/1
  Mux2/1 -> Zone2Z/1
  Mux1/1 -> Zone1Z/1
  <V/1 -> Zone 4/2(<V), Zone 3/2(<V), Zone 2/2(<V), Zone 1/2(<V)
  Complex to Real-Imag/2 -> Mux/2
  Complex to Real-Imag/1 -> Mux/1
  Zone 4/1(TRIP) -> Zone4/1
  Zone 3/1(TRIP) -> Zone3/1
  Zone 2/1(TRIP) -> Zone2/1
  Zone 4/3(Zr) -> Mux4/2
  Zone 4/2(Zm) -> Mux4/1
  Zone 3/3(Zr) -> Mux3/2
  Zone 3/2(Zm) -> Mux3/1
  Zone 2/3(Zr) -> Mux2/2
  Zone 2/2(Zm) -> Mux2/1
  Zone 1/3(Zr) -> Mux1/2
  Zone 1/2(Zm) -> Mux1/1
  Zone 1/1(TRIP) -> Zone1/1
  Mux/1 -> Zone 2/1(Z), Zone 4/1(Z), Zone 3/1(Z), Zone 1/1(Z)
  A-G/1 -> Voltage Current/1

== system OIRT/On-Line Analysis/ZR-1/Impedance Relay Scheme/Fault B-C Measurement ==
  B-C : Inport
  <V : Inport  Port=2
  Complex to Real-Imag : ComplexToRealImag
  Impedance Module : Product  Inputs=*/  SaturateOnIntegerOverflow=on  RndMeth=Zero  InputSameDT=on  OutDataTypeStr=Inherit: Same as first input
  Mux{,1..4} (5 alike) : Mux  Inputs=2
  Voltage Current : Demux  Outputs=2
  Zone 1 : Subsystem  mask(Zone){Xr=ZoneImpedance(1)*sin(LineAngle*pi/180), Rr=ZoneImpedance(1)*cos(LineAngle*pi/180), Td=ZoneTime(1)}
      mask prompts: Xr "Reactance reach [ohm]"; Rr "Resistance reach [ohm]"; Td "Time delay [s]"
  Zone 2 : Subsystem  mask(Zone){Xr=ZoneImpedance(2)*sin(LineAngle*pi/180), Rr=ZoneImpedance(2)*cos(LineAngle*pi/180), Td=ZoneTime(2)}
      mask prompts: Xr "Reactance reach [ohm]"; Rr "Resistance reach [ohm]"; Td "Time delay [s]"
  Zone 3 : Subsystem  mask(Zone){Xr=ZoneImpedance(3)*sin(LineAngle*pi/180), Rr=ZoneImpedance(3)*cos(LineAngle*pi/180), Td=ZoneTime(3)}
      mask prompts: Xr "Reactance reach [ohm]"; Rr "Resistance reach [ohm]"; Td "Time delay [s]"
  Zone 4 : Subsystem  mask(Zone){Xr=ZoneImpedance(4)*sin(LineAngle*pi/180), Rr=ZoneImpedance(4)*cos(LineAngle*pi/180), Td=ZoneTime(4)}
      mask prompts: Xr "Reactance reach [ohm]"; Rr "Resistance reach [ohm]"; Td "Time delay [s]"
  Zone1Z : Terminator
  Zone2Z : Terminator
  Zone3Z : Terminator
  Zone4Z : Terminator
  Zone1 : Outport  InitialOutput=0
  Zone2 : Outport  Port=2  InitialOutput=0
  Zone3 : Outport  Port=3  InitialOutput=0
  Zone4 : Outport  Port=4  InitialOutput=0
  wires:
  B-C/1 -> Voltage Current/1
  Mux/1 -> Zone 1/1(Z), Zone 3/1(Z), Zone 4/1(Z), Zone 2/1(Z)
  Zone 1/1(TRIP) -> Zone1/1
  Zone 1/2(Zm) -> Mux1/1
  Zone 1/3(Zr) -> Mux1/2
  Zone 2/2(Zm) -> Mux2/1
  Zone 2/3(Zr) -> Mux2/2
  Zone 3/2(Zm) -> Mux3/1
  Zone 3/3(Zr) -> Mux3/2
  Zone 4/2(Zm) -> Mux4/1
  Zone 4/3(Zr) -> Mux4/2
  Zone 2/1(TRIP) -> Zone2/1
  Zone 3/1(TRIP) -> Zone3/1
  Zone 4/1(TRIP) -> Zone4/1
  Complex to Real-Imag/1 -> Mux/1
  Complex to Real-Imag/2 -> Mux/2
  <V/1 -> Zone 1/2(<V), Zone 2/2(<V), Zone 3/2(<V), Zone 4/2(<V)
  Mux1/1 -> Zone1Z/1
  Mux2/1 -> Zone2Z/1
  Mux3/1 -> Zone3Z/1
  Mux4/1 -> Zone4Z/1
  Impedance Module/1 -> Complex to Real-Imag/1
  Voltage Current/1 -> Impedance Module/1
  Voltage Current/2 -> Impedance Module/2

== system OIRT/On-Line Analysis/ZR-1/Impedance Relay Scheme/Fault B-G Measurement ==
  B-G : Inport
  <V : Inport  Port=2
  Complex to Real-Imag : ComplexToRealImag
  Impedance Module : Product  Inputs=*/  SaturateOnIntegerOverflow=on  RndMeth=Zero  InputSameDT=on  OutDataTypeStr=Inherit: Same as first input
  Mux{,1..4} (5 alike) : Mux  Inputs=2
  Voltage Current : Demux  Outputs=2
  Zone 1 : Subsystem  mask(Zone){Xr=ZoneImpedance(1)*sin(LineAngle*pi/180), Rr=ZoneImpedance(1)*cos(LineAngle*pi/180), Td=ZoneTime(1)}
      mask prompts: Xr "Reactance reach [ohm]"; Rr "Resistance reach [ohm]"; Td "Time delay [s]"
  Zone 2 : Subsystem  mask(Zone){Xr=ZoneImpedance(2)*sin(LineAngle*pi/180), Rr=ZoneImpedance(2)*cos(LineAngle*pi/180), Td=ZoneTime(2)}
      mask prompts: Xr "Reactance reach [ohm]"; Rr "Resistance reach [ohm]"; Td "Time delay [s]"
  Zone 3 : Subsystem  mask(Zone){Xr=ZoneImpedance(3)*sin(LineAngle*pi/180), Rr=ZoneImpedance(3)*cos(LineAngle*pi/180), Td=ZoneTime(3)}
      mask prompts: Xr "Reactance reach [ohm]"; Rr "Resistance reach [ohm]"; Td "Time delay [s]"
  Zone 4 : Subsystem  mask(Zone){Xr=ZoneImpedance(4)*sin(LineAngle*pi/180), Rr=ZoneImpedance(4)*cos(LineAngle*pi/180), Td=ZoneTime(4)}
      mask prompts: Xr "Reactance reach [ohm]"; Rr "Resistance reach [ohm]"; Td "Time delay [s]"
  Zone1Z : Terminator
  Zone2Z : Terminator
  Zone3Z : Terminator
  Zone4Z : Terminator
  Zone1 : Outport  InitialOutput=0
  Zone2 : Outport  Port=2  InitialOutput=0
  Zone3 : Outport  Port=3  InitialOutput=0
  Zone4 : Outport  Port=4  InitialOutput=0
  wires:
  B-G/1 -> Voltage Current/1
  Mux/1 -> Zone 1/1(Z), Zone 3/1(Z), Zone 4/1(Z), Zone 2/1(Z)
  Zone 1/1(TRIP) -> Zone1/1
  Zone 1/2(Zm) -> Mux1/1
  Zone 1/3(Zr) -> Mux1/2
  Zone 2/2(Zm) -> Mux2/1
  Zone 2/3(Zr) -> Mux2/2
  Zone 3/2(Zm) -> Mux3/1
  Zone 3/3(Zr) -> Mux3/2
  Zone 4/2(Zm) -> Mux4/1
  Zone 4/3(Zr) -> Mux4/2
  Zone 2/1(TRIP) -> Zone2/1
  Zone 3/1(TRIP) -> Zone3/1
  Zone 4/1(TRIP) -> Zone4/1
  Complex to Real-Imag/1 -> Mux/1
  Complex to Real-Imag/2 -> Mux/2
  <V/1 -> Zone 1/2(<V), Zone 2/2(<V), Zone 3/2(<V), Zone 4/2(<V)
  Mux1/1 -> Zone1Z/1
  Mux2/1 -> Zone2Z/1
  Mux3/1 -> Zone3Z/1
  Mux4/1 -> Zone4Z/1
  Impedance Module/1 -> Complex to Real-Imag/1
  Voltage Current/1 -> Impedance Module/1
  Voltage Current/2 -> Impedance Module/2

== system OIRT/On-Line Analysis/ZR-1/Impedance Relay Scheme/Fault C-A Measurement ==
  C-A : Inport
  <V : Inport  Port=2
  Complex to Real-Imag : ComplexToRealImag
  Impedance Module : Product  Inputs=*/  SaturateOnIntegerOverflow=on  RndMeth=Zero  InputSameDT=on  OutDataTypeStr=Inherit: Same as first input
  Mux{,1..4} (5 alike) : Mux  Inputs=2
  Voltage Current : Demux  Outputs=2
  Zone 1 : Subsystem  mask(Zone){Xr=ZoneImpedance(1)*sin(LineAngle*pi/180), Rr=ZoneImpedance(1)*cos(LineAngle*pi/180), Td=ZoneTime(1)}
      mask prompts: Xr "Reactance reach [ohm]"; Rr "Resistance reach [ohm]"; Td "Time delay [s]"
  Zone 2 : Subsystem  mask(Zone){Xr=ZoneImpedance(2)*sin(LineAngle*pi/180), Rr=ZoneImpedance(2)*cos(LineAngle*pi/180), Td=ZoneTime(2)}
      mask prompts: Xr "Reactance reach [ohm]"; Rr "Resistance reach [ohm]"; Td "Time delay [s]"
  Zone 3 : Subsystem  mask(Zone){Xr=ZoneImpedance(3)*sin(LineAngle*pi/180), Rr=ZoneImpedance(3)*cos(LineAngle*pi/180), Td=ZoneTime(3)}
      mask prompts: Xr "Reactance reach [ohm]"; Rr "Resistance reach [ohm]"; Td "Time delay [s]"
  Zone 4 : Subsystem  mask(Zone){Xr=ZoneImpedance(4)*sin(LineAngle*pi/180), Rr=ZoneImpedance(4)*cos(LineAngle*pi/180), Td=ZoneTime(4)}
      mask prompts: Xr "Reactance reach [ohm]"; Rr "Resistance reach [ohm]"; Td "Time delay [s]"
  Zone1Z : Terminator
  Zone2Z : Terminator
  Zone3Z : Terminator
  Zone4Z : Terminator
  Zone1 : Outport  InitialOutput=0
  Zone2 : Outport  Port=2  InitialOutput=0
  Zone3 : Outport  Port=3  InitialOutput=0
  Zone4 : Outport  Port=4  InitialOutput=0
  wires:
  Voltage Current/2 -> Impedance Module/2
  Voltage Current/1 -> Impedance Module/1
  Impedance Module/1 -> Complex to Real-Imag/1
  Mux4/1 -> Zone4Z/1
  Mux3/1 -> Zone3Z/1
  Mux2/1 -> Zone2Z/1
  Mux1/1 -> Zone1Z/1
  <V/1 -> Zone 4/2(<V), Zone 3/2(<V), Zone 2/2(<V), Zone 1/2(<V)
  Complex to Real-Imag/2 -> Mux/2
  Complex to Real-Imag/1 -> Mux/1
  Zone 4/1(TRIP) -> Zone4/1
  Zone 3/1(TRIP) -> Zone3/1
  Zone 2/1(TRIP) -> Zone2/1
  Zone 4/3(Zr) -> Mux4/2
  Zone 4/2(Zm) -> Mux4/1
  Zone 3/3(Zr) -> Mux3/2
  Zone 3/2(Zm) -> Mux3/1
  Zone 2/3(Zr) -> Mux2/2
  Zone 2/2(Zm) -> Mux2/1
  Zone 1/3(Zr) -> Mux1/2
  Zone 1/2(Zm) -> Mux1/1
  Zone 1/1(TRIP) -> Zone1/1
  Mux/1 -> Zone 2/1(Z), Zone 4/1(Z), Zone 3/1(Z), Zone 1/1(Z)
  C-A/1 -> Voltage Current/1

== system OIRT/On-Line Analysis/ZR-1/Impedance Relay Scheme/Fault C-G Measurement ==
  C-G : Inport
  <V : Inport  Port=2
  Complex to Real-Imag : ComplexToRealImag
  Impedance Module : Product  Inputs=*/  SaturateOnIntegerOverflow=on  RndMeth=Zero  InputSameDT=on  OutDataTypeStr=Inherit: Same as first input
  Mux{,1..4} (5 alike) : Mux  Inputs=2
  Voltage Current : Demux  Outputs=2
  Zone 1 : Subsystem  mask(Zone){Xr=ZoneImpedance(1)*sin(LineAngle*pi/180), Rr=ZoneImpedance(1)*cos(LineAngle*pi/180), Td=ZoneTime(1)}
      mask prompts: Xr "Reactance reach [ohm]"; Rr "Resistance reach [ohm]"; Td "Time delay [s]"
  Zone 2 : Subsystem  mask(Zone){Xr=ZoneImpedance(2)*sin(LineAngle*pi/180), Rr=ZoneImpedance(2)*cos(LineAngle*pi/180), Td=ZoneTime(2)}
      mask prompts: Xr "Reactance reach [ohm]"; Rr "Resistance reach [ohm]"; Td "Time delay [s]"
  Zone 3 : Subsystem  mask(Zone){Xr=ZoneImpedance(3)*sin(LineAngle*pi/180), Rr=ZoneImpedance(3)*cos(LineAngle*pi/180), Td=ZoneTime(3)}
      mask prompts: Xr "Reactance reach [ohm]"; Rr "Resistance reach [ohm]"; Td "Time delay [s]"
  Zone 4 : Subsystem  mask(Zone){Xr=ZoneImpedance(4)*sin(LineAngle*pi/180), Rr=ZoneImpedance(4)*cos(LineAngle*pi/180), Td=ZoneTime(4)}
      mask prompts: Xr "Reactance reach [ohm]"; Rr "Resistance reach [ohm]"; Td "Time delay [s]"
  Zone1Z : Terminator
  Zone2Z : Terminator
  Zone3Z : Terminator
  Zone4Z : Terminator
  Zone1 : Outport  InitialOutput=0
  Zone2 : Outport  Port=2  InitialOutput=0
  Zone3 : Outport  Port=3  InitialOutput=0
  Zone4 : Outport  Port=4  InitialOutput=0
  wires:
  Voltage Current/2 -> Impedance Module/2
  Voltage Current/1 -> Impedance Module/1
  Impedance Module/1 -> Complex to Real-Imag/1
  Mux4/1 -> Zone4Z/1
  Mux3/1 -> Zone3Z/1
  Mux2/1 -> Zone2Z/1
  Mux1/1 -> Zone1Z/1
  <V/1 -> Zone 4/2(<V), Zone 3/2(<V), Zone 2/2(<V), Zone 1/2(<V)
  Complex to Real-Imag/2 -> Mux/2
  Complex to Real-Imag/1 -> Mux/1
  Zone 4/1(TRIP) -> Zone4/1
  Zone 3/1(TRIP) -> Zone3/1
  Zone 2/1(TRIP) -> Zone2/1
  Zone 4/3(Zr) -> Mux4/2
  Zone 4/2(Zm) -> Mux4/1
  Zone 3/3(Zr) -> Mux3/2
  Zone 3/2(Zm) -> Mux3/1
  Zone 2/3(Zr) -> Mux2/2
  Zone 2/2(Zm) -> Mux2/1
  Zone 1/3(Zr) -> Mux1/2
  Zone 1/2(Zm) -> Mux1/1
  Zone 1/1(TRIP) -> Zone1/1
  Mux/1 -> Zone 2/1(Z), Zone 4/1(Z), Zone 3/1(Z), Zone 1/1(Z)
  C-G/1 -> Voltage Current/1
